simulink model "Temporal5_2018a"  (R2018a)
settings: Solver=VariableStepAuto  StartTime=0.0  StopTime=1.0  RelTol=1e-3
settings Model: Creator=86188  LastModifiedBy=bzhan

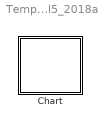
== system Temporal5_2018a ==
  Chart : Stateflow chart  TreatAsAtomicUnit=on

== stateflow chart Temporal5_2018a/Chart ==
  settings: updateMethod=DISCRETE  sampleTime=0.1
  state A
    en:f("en_A");
    x=1;
    du:f("du_A");
    x=x+1;
  state B
    en:f("en_B");
    du:f("du_B");
  (default) -> A
  A -> B : at(4,tick)[x==4]
  B -> A : before(4,tick)
  data: s function_input; x local
  function f(s):
    | function f(s)
    |   fprintf(s+"\n");
